simulink model "main"  (R2019b)
settings: Solver=FixedStepDiscrete  StartTime=0.0  StopTime=180  FixedStep=0.5  RelTol=1e-3
values from neighbouring files (symbols this model uses):
  v_speed = data(:,2)    [dataInput.m]
  v_temp = data(:,3)    [dataInput.m]
  v_time = data(:,1)    [dataInput.m]
settings Model: Creator=yanyx  LastModifiedBy=yanyx

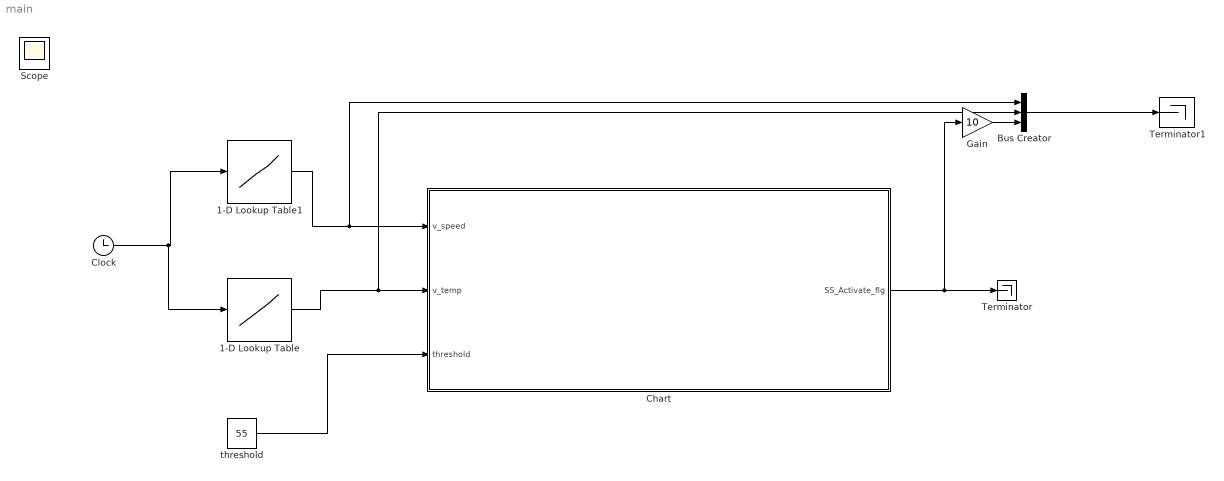
== system main ==
  1-D Lookup Table : Lookup_n-D  NumberOfTableDimensions=1  BreakpointsForDimension1=v_time  Table=v_temp  InternalRulePriority=Speed  RndMeth=Simplest  InputSameDT=on
  1-D Lookup Table1 : Lookup_n-D  NumberOfTableDimensions=1  BreakpointsForDimension1=v_time  Table=v_speed  InternalRulePriority=Speed  RndMeth=Simplest  InputSameDT=on
  Bus Creator : BusCreator  Inputs=3
  Chart : Stateflow chart  BlockKeywords=__PRM__SERIALIZED__DATA__:Stateflow Chart,Stateflow Diagram  TreatAsAtomicUnit=on
  Clock : Clock
  Gain : Gain  Gain=10
  Terminator : Terminator
  Terminator1 : Terminator
  threshold : Constant  Value=55
  Scope : Scope
  wires:
  Clock/1 -> 1-D Lookup Table/1, 1-D Lookup Table1/1
  1-D Lookup Table1/1 -> Bus Creator/1, Chart/1(v_speed)
  1-D Lookup Table/1 -> Bus Creator/2, Chart/2(v_temp)
  threshold/1 -> Chart/3(threshold)
  Chart/1(SS_Activate_flg) -> Gain/1, Terminator/1
  Gain/1 -> Bus Creator/3
  Bus Creator/1 -> Terminator1/1

== stateflow chart main/Chart ==
  state SS_disabled
    entry:
    SS_Activate_flg=0;
  state SS_enabled
    entry:
    SS_Activate_flg=1;
  (default) -> SS_disabled
  SS_enabled -> SS_disabled : [(v_speed >0.5)||(v_temp<threshold)]
  SS_disabled -> SS_enabled : [(v_speed<0.5)&&(v_temp>threshold)]
  data: v_speed input; v_temp input; threshold input; SS_Activate_flg output
